simulink model "EV3robot_model"  (R2016b)
settings: Solver=FixedStepAuto  StartTime=0.0  StopTime=20  RelTol=1e-3  EnableMultiTasking=on
undefined symbols (not defined in the file or in its folder): COLden, COLnum, CPden, CPnum, DiscIntNeverNeededParam, Kc, Km, SqWaveFreq, ThDotRef, Tm, Vm
libraries: legoev3lib x7
settings Model: SimulationMode=external  ExtModeTrigDuration=2  Creator=mwcant  LastModifiedBy=mwcant
settings SolverCC: PositivePriorityOrder=on
settings OptimizationCC: MaxStackSize=64
settings DebuggingCC: ParameterTunabilityLossMsg=error
settings HardwareCC: ProdBitPerPointer=32  ProdBitPerSizeT=32  ProdBitPerPtrDiffT=32  ProdLargestAtomicInteger=Long  ProdWordSize=32  ProdHWDeviceType=ARM Compatible->ARM 9
settings RTWCC: SystemTargetFile=ert.tlc  HardwareBoard=LEGO MINDSTORMS EV3  TLCOptions="-aInlineSetEventsForThisBaseRateFcn=TLC_FALSE -aSuppressMultiTaskScheduler=TLC_FALSE  -aRateBasedStepFcn=0"  TemplateMakefile=ert_default_tmf  Description=Embedded Coder  GenerateReport=on  Toolchain=Sourcery G++ Lite v2009q3  IncludeHyperlinkInReport=on  LaunchReport=on  GenerateTraceInfo=on  GenerateTraceReport=on  GenerateTraceReportSl=on  GenerateTraceReportSf=on  GenerateTraceReportEml=on
settings CodeAppCC: ForceParamTrailComments=on  IgnoreCustomStorageClasses=off  OperatorAnnotations=on  SimulinkDataObjDesc=on  SFDataObjDesc=on  MATLABFcnDesc=on  InsertBlockDesc=on  MATLABSourceComments=on
settings ERTTargetCC: SupportContinuousTime=on  SupportVariableSizeSignals=on  ExtMode=on  ExtModeMexArgs='192.168.1.19' 0 17725

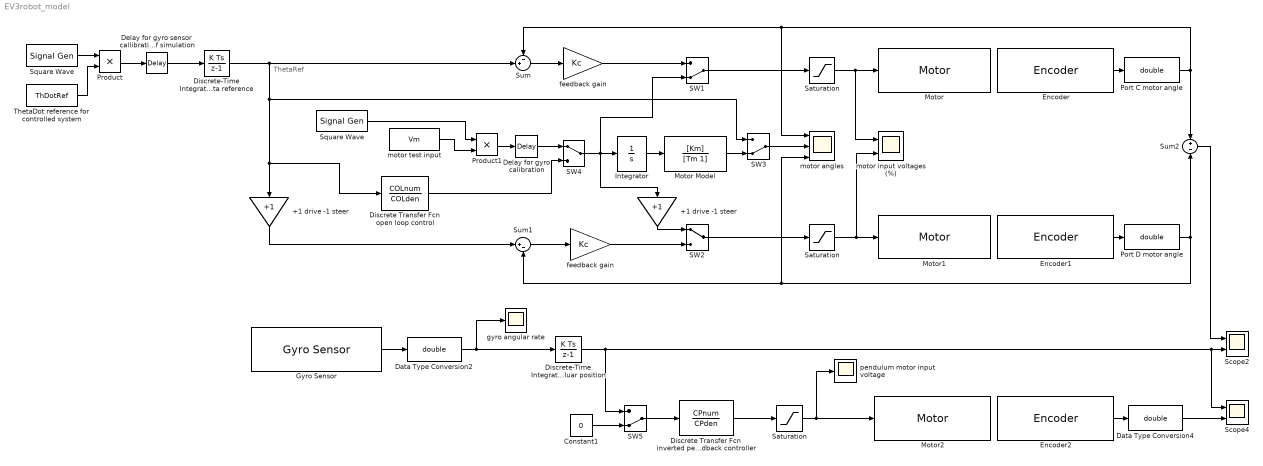
== system EV3robot_model ==
  note: ThetaRef
  "  Saturation" : Saturate  UpperLimit=100  LowerLimit=-100
  +1 drive -1 steer : Gain  Gain=+1
  "+1 drive -1 steer " : Gain  Gain=+1
  Constant1 : Constant  Value=0
  Data Type Conversion2 : DataTypeConversion  OutDataTypeStr=double
  Data Type Conversion4 : DataTypeConversion  OutDataTypeStr=double
  Delay for gyro calibration : TransportDelay  DelayTime=2  FixedBuffer=on
  "Delay for gyro sensor callibration at start of simulation " : TransportDelay  DelayTime=2  FixedBuffer=on
  Discrete Transfer Fcn inverted pendulum feedback controller : DiscreteTransferFcn  Numerator=CPnum  Denominator=CPden
  Discrete Transfer Fcn open loop control : DiscreteTransferFcn  Numerator=COLnum  Denominator=COLden
  Discrete-Time Integrator to convert ThetaDot reference to a Theta reference : DiscreteIntegrator  InitialConditionSetting=State (most efficient)  SampleTime=-1  ICPrevOutput=DiscIntNeverNeededParam  ICPrevScaledInput=DiscIntNeverNeededParam
  Discrete-Time Integrator to convert gyro rate to angluar position : DiscreteIntegrator  InitialConditionSetting=State (most efficient)  SampleTime=-1  ICPrevOutput=DiscIntNeverNeededParam  ICPrevScaledInput=DiscIntNeverNeededParam
  Encoder : legoev3lib/Encoder  portNumber=C  opMode=No reset  sampleTime=Ts
  Encoder1 : legoev3lib/Encoder  portNumber=D  opMode=No reset  sampleTime=Ts
  Encoder2 : legoev3lib/Encoder  portNumber=A  opMode=No reset  sampleTime=Ts
  Gyro Sensor : legoev3lib/Gyro Sensor  portNumber=1  sampleTime=Ts
  Integrator : Integrator
  Motor : legoev3lib/Motor  sportNumber=C  sstopAction=Brake
  Motor Model : TransferFcn  Numerator=[Km]  Denominator=[Tm 1]
  Motor1 : legoev3lib/Motor  sportNumber=D  sstopAction=Brake
  Motor2 : legoev3lib/Motor  sportNumber=A  sstopAction=Brake
  Port C motor angle : DataTypeConversion  OutDataTypeStr=double
  Port D motor angle : DataTypeConversion  OutDataTypeStr=double
  Product : Product
  Product1 : Product
  SW1 : ManualSwitch  CurrentSetting=0
  SW2 : ManualSwitch
  SW3 : ManualSwitch  CurrentSetting=0
  SW4 : ManualSwitch
  "SW5 " : ManualSwitch  CurrentSetting=0
  Saturation : Saturate  UpperLimit=100  LowerLimit=-100
  "Saturation " : Saturate  UpperLimit=100  LowerLimit=-100
  Scope2 : Scope  NumInputPorts=2
  Scope4 : Scope  NumInputPorts=2
  Square Wave : SignalGenerator  WaveForm=square  Frequency=SqWaveFreq
  "Square Wave " : SignalGenerator  WaveForm=square  Frequency=SqWaveFreq
  Sum : Sum  Inputs=-+|
  Sum1 : Sum  Inputs=|+-
  Sum2 : Sum  Inputs=+-
  ThetaDot reference for controlled system : Constant  Value=ThDotRef
  feedback gain : Gain  Gain=Kc
  "feedback gain " : Gain  Gain=Kc
  gyro angular rate : Scope
  motor angles : Scope  NumInputPorts=3
  "motor input voltages (%) " : Scope  NumInputPorts=2
  motor test input : Constant  Value=Vm
  pendulum motor input voltage : Scope
  wires:
  Sum/1 -> feedback gain/1
  Port C motor angle/1 -> Sum2/1, Sum/1, motor angles/1
  Encoder1/1 -> Port D motor angle/1
  Sum1/1 -> "feedback gain "/1
  Port D motor angle/1 -> Sum1/2, motor angles/3, Sum2/2
  Gyro Sensor/1 -> Data Type Conversion2/1
  +1 drive -1 steer/1 -> Sum1/1
  Data Type Conversion2/1 -> Discrete-Time Integrator to convert gyro rate to angluar position/1, gyro angular rate/1
  Saturation/1 -> "motor input voltages (%) "/1, Motor/1
  "Saturation "/1 -> "motor input voltages (%) "/2, Motor1/1
  Discrete-Time Integrator to convert gyro rate to angluar position/1 -> Scope4/1, Scope2/2, "SW5 "/1
  SW2/1 -> "Saturation "/1
  "feedback gain "/1 -> SW2/2
  SW1/1 -> Saturation/1
  feedback gain/1 -> SW1/1
  Encoder/1 -> Port C motor angle/1
  Square Wave/1 -> Product/1
  Product/1 -> "Delay for gyro sensor callibration at start of simulation "/1
  Sum2/1 -> Scope2/1
  Encoder2/1 -> Data Type Conversion4/1
  Discrete Transfer Fcn inverted pendulum feedback controller/1 -> "  Saturation"/1
  "  Saturation"/1 -> Motor2/1, pendulum motor input voltage/1
  "SW5 "/1 -> Discrete Transfer Fcn inverted pendulum feedback controller/1
  Constant1/1 -> "SW5 "/2
  "Delay for gyro sensor callibration at start of simulation "/1 -> Discrete-Time Integrator to convert ThetaDot reference to a Theta reference/1
  ThetaDot reference for controlled system/1 -> Product/2
  motor test input/1 -> Product1/2
  "Square Wave "/1 -> Product1/1
  Product1/1 -> Delay for gyro calibration/1
  Integrator/1 -> Motor Model/1
  SW4/1 -> Integrator/1, SW1/2, "+1 drive -1 steer "/1
  Motor Model/1 -> SW3/2
  SW3/1 -> motor angles/2
  Data Type Conversion4/1 -> Scope4/2
  "+1 drive -1 steer "/1 -> SW2/1
  Delay for gyro calibration/1 -> SW4/1
  Discrete-Time Integrator to convert ThetaDot reference to a Theta reference/1 -> SW3/1, Discrete Transfer Fcn open loop control/1, +1 drive -1 steer/1, Sum/2
  Discrete Transfer Fcn open loop control/1 -> SW4/2
